simulink model "playback_4khz"  (R2018b)
settings: configuration reference "Configuration4khzPlayback" (kept outside this file)
values from neighbouring files (symbols this model uses):
  sample_time = 0.0005    [ElmoIncremental.m]
undefined symbols (not defined in the file or in its folder): elmo_sample_time, time_1000_recorded, time_4000_recorded
libraries: simulink x2
settings Model: Creator=wmartin  LastModifiedBy=AtriasUser2
settings ConfigSetRef: SourceLocation=Base Workspace

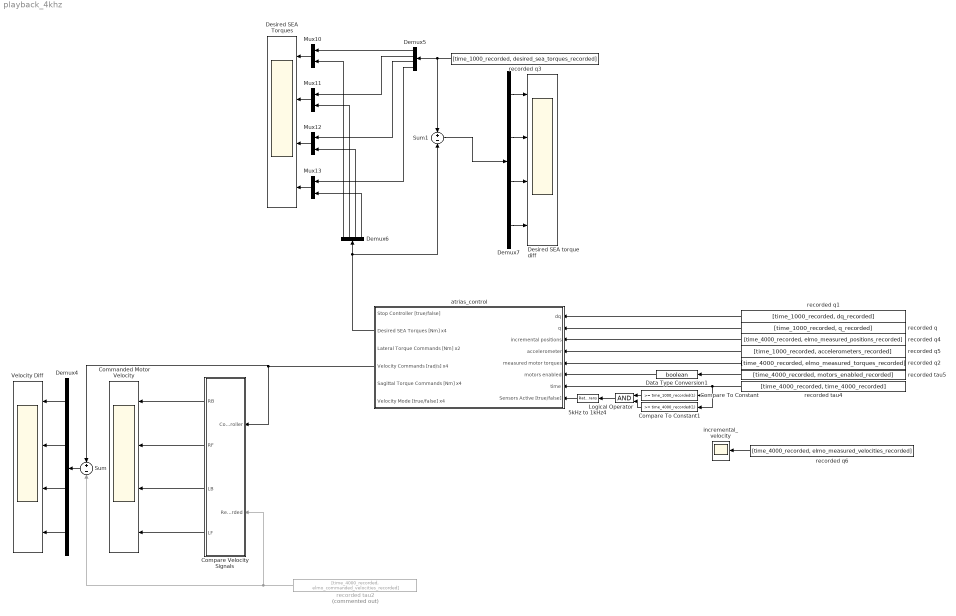
== system playback_4khz ==
  5kHz to 1kHz4 : RateTransition  Deterministic=off  OutPortSampleTime=sample_time
  Commanded Motor Velocity : Scope  NumInputPorts=4
  Compare To Constant : simulink/Logic and Bit Operations/Compare To Constant  relop=>=  const=time_1000_recorded(1)  OutDataTypeStr=boolean
  Compare To Constant1 : simulink/Logic and Bit Operations/Compare To Constant  relop=>=  const=time_4000_recorded(1)  OutDataTypeStr=boolean
  Compare Velocity Signals : Subsystem
  Data Type Conversion1 : DataTypeConversion  OutDataTypeStr=boolean
  Demux{4..7} (4 alike) : Demux
  Desired SEA Torques : Scope  NumInputPorts=4
  Desired SEA torque diff : Scope  NumInputPorts=4
  Logical Operator : Logic  AllPortsSameDT=off  OutDataTypeStr=boolean
  Mux{10..13} (4 alike) : Mux  Inputs=2
  Sum : Sum  Inputs=+-
  Sum1 : Sum  Inputs=+-
  Velocity Diff : Scope  NumInputPorts=4
  atrias_control : Subsystem
  incremental_velocity : Scope
  recorded q : FromWorkspace  VariableName=[time_1000_recorded, q_recorded]  OutDataTypeStr=double  SampleTime=sample_time  Interpolate=off  OutputAfterFinalValue=Holding final value
  recorded q1 : FromWorkspace  VariableName=[time_1000_recorded, dq_recorded]  OutDataTypeStr=double  SampleTime=sample_time  Interpolate=off  OutputAfterFinalValue=Holding final value
  recorded q2 : FromWorkspace  VariableName=[time_4000_recorded, elmo_measured_torques_recorded]  OutDataTypeStr=double  SampleTime=elmo_sample_time  Interpolate=off  OutputAfterFinalValue=Holding final value
  recorded q3 : FromWorkspace  VariableName=[time_1000_recorded, desired_sea_torques_recorded]  OutDataTypeStr=double  SampleTime=sample_time  Interpolate=off  OutputAfterFinalValue=Holding final value
  recorded q4 : FromWorkspace  VariableName=[time_4000_recorded, elmo_measured_positions_recorded]  OutDataTypeStr=double  SampleTime=elmo_sample_time  Interpolate=off  OutputAfterFinalValue=Holding final value
  recorded q5 : FromWorkspace  VariableName=[time_1000_recorded, accelerometers_recorded]  OutDataTypeStr=double  SampleTime=sample_time  Interpolate=off  OutputAfterFinalValue=Holding final value
  recorded q6 : FromWorkspace  VariableName=[time_4000_recorded, elmo_measured_velocities_recorded]  OutDataTypeStr=double  SampleTime=elmo_sample_time  Interpolate=off  OutputAfterFinalValue=Holding final value
  recorded tau2 : FromWorkspace  Commented=on  VariableName=[time_4000_recorded, elmo_commanded_velocities_recorded]  OutDataTypeStr=double  SampleTime=elmo_sample_time  Interpolate=off  OutputAfterFinalValue=Holding final value
  recorded tau4 : FromWorkspace  VariableName=[time_4000_recorded, time_4000_recorded]  OutDataTypeStr=double  SampleTime=elmo_sample_time  Interpolate=off  OutputAfterFinalValue=Holding final value
  recorded tau5 : FromWorkspace  VariableName=[time_4000_recorded, motors_enabled_recorded]  OutDataTypeStr=double  SampleTime=elmo_sample_time  Interpolate=off  OutputAfterFinalValue=Holding final value
  wires:
  Compare Velocity Signals/1(RB) -> Commanded Motor Velocity/1
  Compare Velocity Signals/2(RF) -> Commanded Motor Velocity/2
  Compare Velocity Signals/3(LB) -> Commanded Motor Velocity/3
  Compare Velocity Signals/4(LF) -> Commanded Motor Velocity/4
  Demux4/4 -> Velocity Diff/4
  Demux4/3 -> Velocity Diff/3
  Demux4/2 -> Velocity Diff/2
  Demux4/1 -> Velocity Diff/1
  Mux10/1 -> Desired SEA Torques/1
  Mux11/1 -> Desired SEA Torques/2
  Mux12/1 -> Desired SEA Torques/3
  Mux13/1 -> Desired SEA Torques/4
  Demux5/2 -> Mux11/1
  Demux5/3 -> Mux12/1
  Demux5/4 -> Mux13/1
  Demux6/1 -> Mux10/2
  Demux6/2 -> Mux11/2
  Demux6/3 -> Mux12/2
  Demux6/4 -> Mux13/2
  recorded q3/1 -> Demux5/1, Sum1/1
  Demux5/1 -> Mux10/1
  atrias_control/2(Desired SEA Torques [Nm] x4) -> Sum1/2, Demux6/1
  Demux7/3 -> Desired SEA torque diff/3
  Demux7/2 -> Desired SEA torque diff/2
  Demux7/1 -> Desired SEA torque diff/1
  Demux7/4 -> Desired SEA torque diff/4
  Sum1/1 -> Demux7/1
  recorded q/1 -> atrias_control/2(q)
  recorded tau5/1 -> Data Type Conversion1/1
  recorded q4/1 -> atrias_control/3(incremental positions)
  Data Type Conversion1/1 -> atrias_control/6(motors enabled)
  recorded q2/1 -> atrias_control/5(measured motor torques)
  recorded q5/1 -> atrias_control/4(accelerometer)
  recorded q1/1 -> atrias_control/1(dq)
  Compare To Constant1/1 -> Logical Operator/2
  Compare To Constant/1 -> Logical Operator/1
  Logical Operator/1 -> 5kHz to 1kHz4/1
  Sum/1 -> Demux4/1
  atrias_control/4(Velocity Commands [rad/s] x4) -> Compare Velocity Signals/1(Controller), Sum/1
  recorded tau2/1 -> Compare Velocity Signals/2(Recorded), Sum/2
  5kHz to 1kHz4/1 -> atrias_control/8(Sensors Active [true/false])
  recorded tau4/1 -> atrias_control/7(time), Compare To Constant1/1, Compare To Constant/1
  recorded q6/1 -> incremental_velocity/1

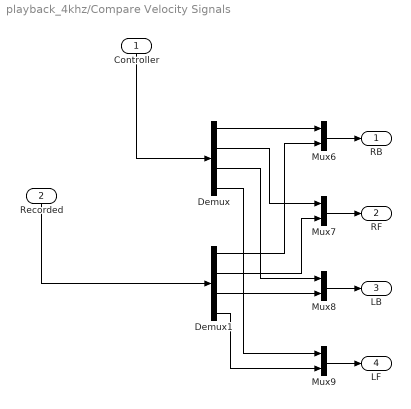
== system playback_4khz/Compare Velocity Signals ==
  Controller : Inport
  Recorded : Inport  Port=2
  Demux : Demux
  Demux1 : Demux
  Mux{6..9} (4 alike) : Mux  Inputs=2
  RB : Outport
  RF : Outport  Port=2
  LB : Outport  Port=3
  LF : Outport  Port=4
  wires:
  Demux/3 -> Mux8/1
  Demux/2 -> Mux7/1
  Demux1/1 -> Mux6/2
  Demux/1 -> Mux6/1
  Demux/4 -> Mux9/1
  Demux1/4 -> Mux9/2
  Recorded/1 -> Demux1/1
  Demux1/2 -> Mux7/2
  Controller/1 -> Demux/1
  Demux1/3 -> Mux8/2
  Mux6/1 -> RB/1
  Mux7/1 -> RF/1
  Mux8/1 -> LB/1
  Mux9/1 -> LF/1

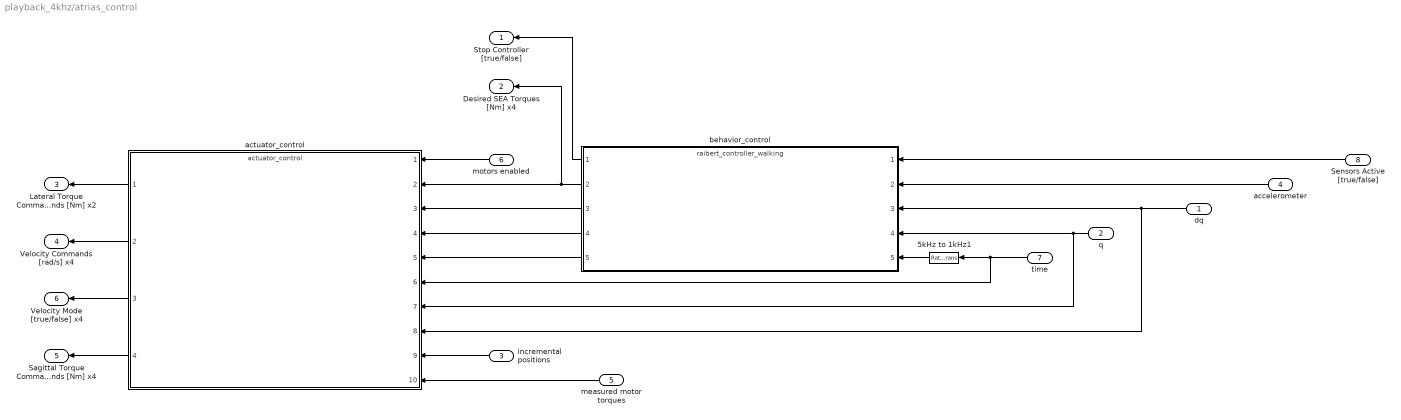
== system playback_4khz/atrias_control ==
  dq : Inport  OutDataTypeStr=double  PortDimensions=13  SampleTime=[0.001,0]
  q : Inport  Port=2  OutDataTypeStr=double  PortDimensions=13  SampleTime=[0.001,0]
  incremental positions : Inport  Port=3  OutDataTypeStr=double  PortDimensions=4  SampleTime=[0.00025000000000000001,0]
  accelerometer : Inport  Port=4  OutDataTypeStr=double  PortDimensions=3  SampleTime=[0.001,0]
  measured motor torques : Inport  Port=5  OutDataTypeStr=double  PortDimensions=4  SampleTime=[0.00025000000000000001,0]
  motors enabled : Inport  Port=6  OutDataTypeStr=boolean  PortDimensions=1  SampleTime=[0.00025000000000000001,0]
  time : Inport  Port=7  OutDataTypeStr=double  PortDimensions=1  SampleTime=elmo_sample_time
  Sensors Active [true/false] : Inport  Port=8  PortDimensions=1  SampleTime=elmo_sample_time
  5kHz to 1kHz1 : RateTransition  Deterministic=off  OutPortSampleTime=sample_time
  actuator_control : ModelReference  ModelNameDialog=actuator_control  SimulationMode=Normal  ModelReferenceVersion=1.1706
  behavior_control : ModelReference  ModelNameDialog=raibert_controller_walking  SimulationMode=Normal  ModelReferenceVersion=1.9533
  Stop Controller [true/false] : Outport  OutDataTypeStr=boolean  PortDimensions=1  SampleTime=[0.001,0]  InitialOutput=[0 0 0 0]
  Desired SEA Torques [Nm] x4 : Outport  Port=2  OutDataTypeStr=double  PortDimensions=4  SampleTime=[0.001,0]  InitialOutput=[0 0 0 0]
  Lateral Torque Commands [Nm] x2 : Outport  Port=3  OutDataTypeStr=double  PortDimensions=2  SampleTime=[0.00025000000000000001,0]  InitialOutput=[0 0]
  Velocity Commands [rad/s] x4 : Outport  Port=4  OutDataTypeStr=double  PortDimensions=4  SampleTime=[0.00025000000000000001,0]  InitialOutput=[0 0 0 0]
  Sagittal Torque Commands [Nm] x4 : Outport  Port=5  OutDataTypeStr=double  PortDimensions=4  SampleTime=[0.00025000000000000001,0]  InitialOutput=[0 0 0 0]
  Velocity Mode [true/false] x4 : Outport  Port=6  OutDataTypeStr=boolean  PortDimensions=4  SampleTime=[0.00025000000000000001,0]  InitialOutput=[true true true true]
  wires:
  actuator_control/4 -> Sagittal Torque Commands [Nm] x4/1
  actuator_control/2 -> Velocity Commands [rad/s] x4/1
  actuator_control/3 -> Velocity Mode [true/false] x4/1
  Sensors Active [true/false]/1 -> behavior_control/1
  time/1 -> actuator_control/6, 5kHz to 1kHz1/1
  q/1 -> actuator_control/7, behavior_control/4
  behavior_control/2 -> Desired SEA Torques [Nm] x4/1, actuator_control/2
  dq/1 -> actuator_control/8, behavior_control/3
  actuator_control/1 -> Lateral Torque Commands [Nm] x2/1
  accelerometer/1 -> behavior_control/2
  motors enabled/1 -> actuator_control/1
  5kHz to 1kHz1/1 -> behavior_control/5
  behavior_control/1 -> Stop Controller [true/false]/1
  behavior_control/3 -> actuator_control/3
  behavior_control/4 -> actuator_control/4
  behavior_control/5 -> actuator_control/5
  incremental positions/1 -> actuator_control/9
  measured motor torques/1 -> actuator_control/10
